simulink model "rrmc"  (R2020a)
settings: Solver=ode45  StartTime=0.0  StopTime=5.0  RelTol=1e-3  EnableMultiTasking=on
undefined symbols (not defined in the file or in its folder): DiscIntNeverNeededParam
libraries: roblocks x4, simulink x1
settings Model: ExtModeAutoUpdateStatusClock=off  Creator=pic  LastModifiedBy=mluser
settings DataIOCC: SaveFormat=Array  SignalLoggingSaveFormat=ModelDataLogs  SignalLoggingName=sigsOut
settings OptimizationCC: ExpressionDepthLimit=2147483647  LifeSpan=inf
settings DebuggingCC: SaveWithParameterizedLinksMsg=none  UnderspecifiedInitializationDetection=Classic  MergeDetectMultiDrivingBlocksExec=none  SignalResolutionControl=TryResolveAllWithWarning  MultiTaskDSMMsg=warning  MultiTaskCondExecSysMsg=none  FcnCallInpInsideContextMsg=warning  StateNameClashWarn=warning  SFUnexpectedBacktrackingDiag=warning  SFNoUnconditionalDefaultTransitionDiag=warning  SFExecutionAtInitializationDiag=none  ArithmeticOperatorsInVariantConditions=warning
settings HardwareCC: ProdBitPerPointer=32  ProdBitPerSizeT=32  ProdBitPerPtrDiffT=32  ProdLargestAtomicFloat=None  ProdIntDivRoundTo=Undefined  ProdEndianess=Unspecified  ProdWordSize=32  ProdHWDeviceType=32-bit Generic  TargetUnknown=on
settings ModelReferenceCC: PropagateSignalLabelsOutOfModel=off
settings SFSimCC: SimUseLocalCustomCode=off  CustomCodeUndefinedFunction=UseInterfaceOnly
settings RTWCC: RTWUseLocalCustomCode=off
settings CodeAppCC: StateflowObjectComments=on
settings GRTTargetCC: TargetLangStandard=C89/C90 (ANSI)  CombineOutputUpdateFcns=off  GRTInterface=on
settings ConfigComp: CovMetricSettings=dw  CovHtmlReporting=on  CovSaveCumulativeToWorkspaceVar=on  CovSaveSingleToWorkspaceVar=on  CovExternalEMLEnable=off

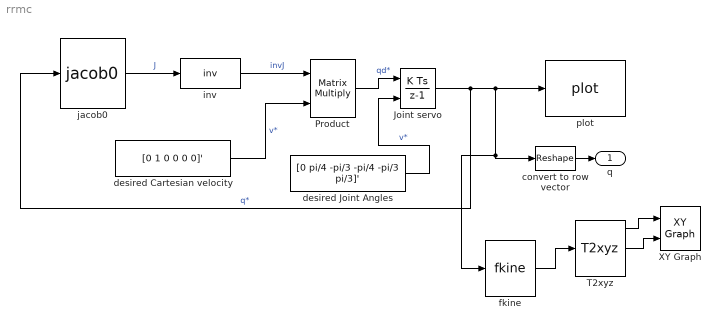
== system rrmc ==
  Joint servo : DiscreteIntegrator  InitialConditionSource=external  InitialCondition=qn'  SampleTime=0.05  ICPrevOutput=DiscIntNeverNeededParam  ICPrevScaledInput=DiscIntNeverNeededParam
  Product : Product  Multiplication=Matrix(*)  SaturateOnIntegerOverflow=on  OutDataTypeStr=Inherit: Same as first input
  T2xyz : roblocks/Transform Conversion/T2xyz
  XY Graph : simulink/Sinks/XY Graph  xmin=-1  xmax=30  ymin=-1  ymax=30  st=-1
  convert to row vector : Reshape  OutputDimensionality=Customize  OutputDimensions=6
  desired Cartesian velocity : Constant  Value=[0 1 0 0 0 0]'  VectorParams1D=off
  desired Joint Angles : Constant  Value=[0 pi/4 -pi/3 -pi/4 -pi/3 pi/3]'  VectorParams1D=off
  fkine : roblocks/Kinematics/fkine  robot=planar3d
  inv : MATLABFcn  MATLABFcn=inv  Output1D=off
  "jacob0 " : roblocks/Kinematics/jacob0   robot=planar3d
  plot : roblocks/Robot Graphics/plot  robot=planar3d  fps=25  holdplot=on
  q : Outport
  wires:
  "jacob0 "/1 -> inv/1  "J"
  Product/1 -> Joint servo/1  "qd*"
  Joint servo/1 -> "jacob0 "/1, plot/1, fkine/1, convert to row vector/1  "q*"
  inv/1 -> Product/1  "invJ"
  desired Cartesian velocity/1 -> Product/2  "v*"
  convert to row vector/1 -> q/1
  desired Joint Angles/1 -> Joint servo/2  "v*"
  fkine/1 -> T2xyz/1
  T2xyz/1 -> XY Graph/1
  T2xyz/2 -> XY Graph/2
